simulink model "Solucionproblema"  (R2020b)
settings: Solver=VariableStepAuto  StartTime=0.0  StopTime=5.0  RelTol=1e-3
settings Model: Creator=usuario  LastModifiedBy=usuario

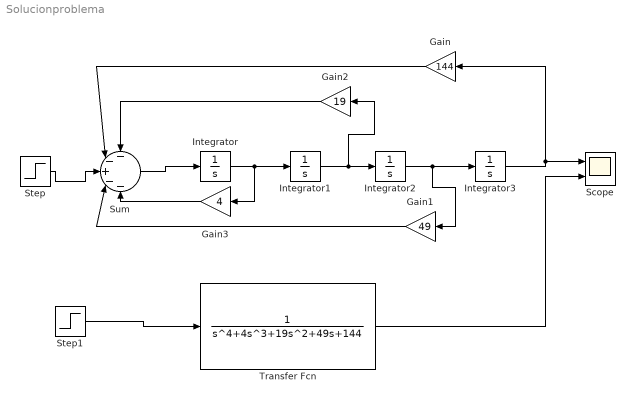
== system Solucionproblema ==
  Gain : Gain  Gain=144
  Gain1 : Gain  Gain=49
  Gain2 : Gain  Gain=19
  Gain3 : Gain  Gain=4
  Integrator{,1..3} (4 alike) : Integrator
  Scope : Scope  NumInputPorts=2
  Step : Step  Time=0  SampleTime=0
  Step1 : Step  Time=0  SampleTime=0
  Sum : Sum  Inputs=--+--
  Transfer Fcn : TransferFcn  Denominator=[1 4 19 49 144]
  wires:
  Integrator2/1 -> Gain1/1, Integrator3/1
  Integrator1/1 -> Gain2/1, Integrator2/1
  Integrator/1 -> Gain3/1, Integrator1/1
  Step/1 -> Sum/3
  Sum/1 -> Integrator/1
  Integrator3/1 -> Scope/1, Gain/1
  Gain/1 -> Sum/2
  Gain1/1 -> Sum/4
  Gain2/1 -> Sum/1
  Gain3/1 -> Sum/5
  Step1/1 -> Transfer Fcn/1
  Transfer Fcn/1 -> Scope/2
